simulink model "sgMdl_IO325_IO336_AnalogLoopback"  (R2024b)
settings: Solver=FixedStepAuto  StartTime=0.0  StopTime=inf  RelTol=1e-3
undefined symbols (not defined in the file): Pull, pull, up
libraries: speedgoatlib_fpga_analog_io x3, slrealtimeloglib x2, speedgoatlib_fpga x1
Description:
  | IO325 & IO336 - Analog Loopback
settings Model: ModifiedByFormat=Speedgoat  SimulationMode=external  ExtModeTrigDuration=100000  Creator=Speedgoat  LastModifiedBy=Speedgoat
settings SolverCC: ConcurrentTasks=on  PositivePriorityOrder=on
settings DataIOCC: SaveFormat=StructureWithTime
settings OptimizationCC: BlockReduction=off  OptimizeBlockIOStorage=off  BufferReuse=off  ReuseModelBlockBuffer=off
settings DebuggingCC: UnderspecifiedInitializationDetection=Classic  MergeDetectMultiDrivingBlocksExec=none  TasksWithSamePriorityMsg=none
settings HardwareCC: ProdBitPerLong=64  ProdLongLongMode=on  ProdHWDeviceType=Intel->x86-64 (Linux 64)
settings ModelReferenceCC: EnableRefExpFcnMdlSchedulingChecks=on  PropagateSignalLabelsOutOfModel=off
settings RTWCC: Description=Speedgoat Real-Time Target Machine  SystemTargetFile=speedgoat.tlc  TemplateMakefile=slrealtime_default_tmf  PostCodeGenCommand=sg.model.build.makeCfg(bdroot, buildInfo);  Toolchain=Simulink Real-Time Toolchain  BuildConfiguration=Faster Runs  TargetLang=C++  GPUComputeCapability=3.5
settings SimulinkRealTimeTargetCC: SubcomponentCodeInterfacePackaging=Reusable function  InstructionSetFMA=off  LogToMDFFile=off  SLRTFileLogMaxRuns=10
settings ConfigComp: CovBoundaryAbsTol=1.0e-5

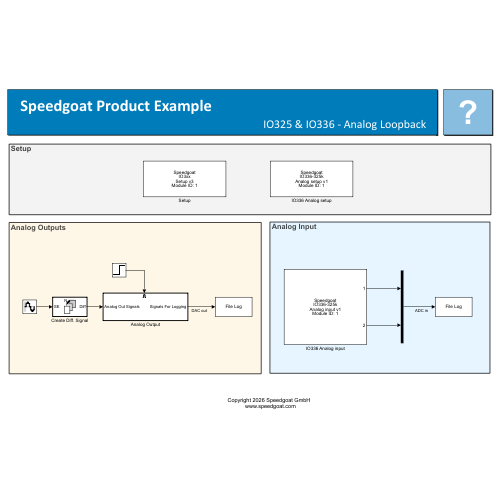
[thumbnail: Simulink's stored preview of the top-level diagram]
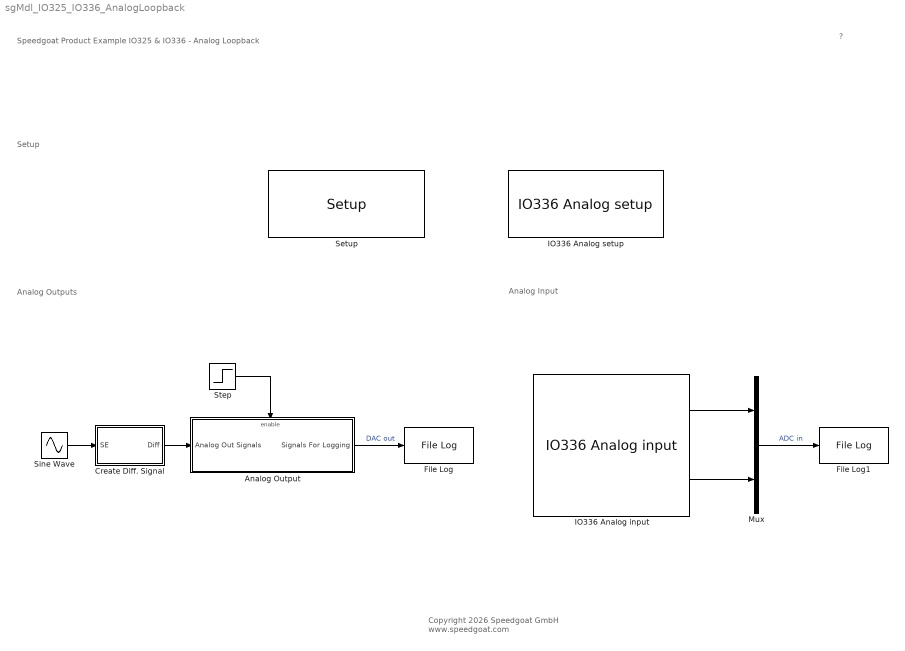
== system sgMdl_IO325_IO336_AnalogLoopback ==
  note: Analog Outputs
  note: Analog Input
  note: Setup
  note: Speedgoat Product Example
      | IO325 & IO336 - Analog Loopback
  note: ?
  note: Copyright 2026 Speedgoat GmbH
      |  www.speedgoat.com
  Analog Output : Subsystem
  Create Diff. Signal : Subsystem  TreatAsAtomicUnit=on
  File Log : slrealtimeloglib/File Log  decimation=1  inputProcessing=Elements as channels (sample based)
  File Log1 : slrealtimeloglib/File Log  decimation=1  inputProcessing=Elements as channels (sample based)
  IO336 Analog input : speedgoatlib_fpga_analog_io/IO336/IO336 Analog input  id=1  parSampleTime=1e-3  pciSlot=[-1,-1]  parAiChannels=[1 2]  parAiChannelsStreamed=[1 2]  parAiTriggerMode=[1 1]  parAiReadPrevValue=0  parAiEnableFrame=0  parAiVoltageRange=[0 3 3 3 3 3 3 3]  parAdcCoupling=[1 1 1 1]  parAdcContSampling=0  parAdcDmaEnable=0  parAdcActiveDmaDevices=[1 1 1 1]  parAiFrameSize=100
      settings: SourceProductName=Analog IO
  IO336 Analog setup : speedgoatlib_fpga_analog_io/IO336/IO336 Analog setup  id=1  parEnableCodeModule1=off  parEnableCodeModule2=off  parEnableCodeModule3=off  parEnableCodeModule4=off  parEnableCodeModule5=off  parEnableCodeModule6=off  parEnableCodeModule7=off  parEnableCodeModule8=off  parAdcEnableIndividualTrigger=off  parAdcTriggerMode1=Model Step  parAdcSampleRate1=0  parAdcDioTriggerChannel1=1  parAdcInternalTrigger1=<empty>  parAdcOversampling1=None  parAdcTriggerMode2=Model Step  parAdcSampleRate2=0  parAdcDioTriggerChannel2=1  parAdcInternalTrigger2=<empty>  parAdcOversampling2=None  parAdcReadPrevValueIndividualTrigger=off  parAdcEnableFrame=off  parAdcTriggerMode=Model Step  parAdcReadPrevValue=off  parAdcSampleRate=100e3  parAdcDioTriggerChannel=1  parAdcInternalTrigger=<empty>  parAdcOversampling=None  parAdcTriggerResolution=1e-08  parAdcSampleRateFrame=100e3  parAdcFrameSize=100  parAdcSampleTime=0.1  parDacTriggerMode=Model Step  parDacInternalTrigger=<empty>  parDacDioTriggerChannel=0  parDacEnableFrame=on  dacUsesTimer=on  parDacFifoThreshold=100  parDacTriggerResolution=1e-08  parDacSampleRate=1e6  parDacFrameSize=100  parDacSampleTime=0.1  parAdcChannel1=on  parAdcChannel2=on  parAdcChannel3=off  parAdcChannel4=off  parAdcChannel5=off  parAdcChannel6=off  parAdcChannel7=off  parAdcChannel8=off  parVoltageRangePerChannelEn1=off  parAdcRangeAll1=+/- 20V  parAdcRange1=+/- 20V  parAdcRange3=+/- 20V  parAdcRange2=+/- 20V  parAdcRange4=+/- 20V  parAdcChannel9=off  parAdcChannel10=off  parAdcChannel11=off  parAdcChannel12=off  parAdcChannel13=off  parAdcChannel14=off  parAdcChannel15=off  parAdcChannel16=off  parVoltageRangePerChannelEn2=off  parAdcRangeAll2=+/- 20V  parAdcRange5=+/- 20V  parAdcRange7=+/- 20V  parAdcRange6=+/- 20V  parAdcRange8=+/- 20V  parAdcAutoCorrection=on  parDacChannel1=on  parDacChannel2=on  parDacChannel3=on  parDacChannel4=on  parDacChannel5=off  parDacChannel6=off  parDacChannel7=off  parDacChannel8=off  parDacRange1=+-10 V  parDacInitValue1=0.5  parDacReset1=on  parDacRange2=+-10 V  parDacInitValue2=-0.5  parDacReset2=on  parDacRange3=+-10 V  parDacInitValue3=1  parDacReset3=on  parDacRange4=+-10 V  parDacInitValue4=-1  parDacReset4=on  parDacRange5=+-5 V  parDacInitValue5=0  parDacReset5=on  parDacRange6=+-5 V  parDacInitValue6=0  parDacReset6=on  parDacRange7=+-5 V  parDacInitValue7=0  parDacReset7=on  parDacRange8=+-5 V  parDacInitValue8=0  parDacReset8=on  parDacAutoCorrection=on
      settings: SourceProductName=Analog IO
  Mux : Mux  Inputs=2
  Setup : speedgoatlib_fpga/Setup/Setup  board=Please select...  id=1  pciSlot=-1  device_id=1  bitstreamFilePath=C:\SVN\speedgoatlib\releases\10.0.0\product_examples\IO325_IO336  bitstreamFile=Please select...  fpgaFreq=[100000000 100000000]  enableDma=on  rearEnb_1=off  rearIO_1=None  rearEnb_2=off  rearIO_2=None  ProgSpiFlash=off  ProgBPIFlash=off  useFpgaDmaController=off  dmaTrigDropdown=Model Step  dmaTrigSelect=0  dmaStopOnOverload=on  dmaModeSequential=on  dmaModeParallel=off  PullRPort15=pull-up 3.3V  PullRPort31=pull-up 3.3V  PullRPort47=pull-up 3.3V  PullRPort63=pull-up 3.3V  diffLineTermination_1=on  diffLineTermination_2=on  diffLineTermination_3=on  diffLineTermination_4=on  diffLineTermination_5=on  diffLineTermination_6=on  diffLineTermination_7=on  diffLineTermination_8=on  diffLineTermination_9=on  diffLineTermination_10=on  diffLineTermination_11=on  diffLineTermination_12=on  diffLineTermination_13=on  diffLineTermination_14=on  diffLineTermination_15=on  diffLineTermination_16=on  diffLineTermination_17=on  diffLineTermination_18=on  diffLineTermination_19=on  diffLineTermination_20=on  diffLineTermination_21=on  diffLineTermination_22=on  diffLineTermination_23=on  diffLineTermination_24=on  diffLineTermination_25=on  diffLineTermination_26=on  diffLineTermination_27=on  diffLineTermination_28=on  diffLineTermination_29=on  diffLineTermination_30=on  diffLineTermination_31=on  diffLineTermination_32=on  ioVoltageDropDown1=3.3V  pullResistorDropDown1_1=Pull-up  pullResistorDropDown1_2=Pull-up  pullResistorDropDown1_3=Pull-up  pullResistorDropDown1_4=Pull-up  pullResistorDropDown1_5=Pull-up  pullResistorDropDown1_6=Pull-up  pullResistorDropDown1_7=Pull-up  pullResistorDropDown1_8=Pull-up  ttlIsImplementedCheckBox1=off  pullResistorDropDown2=Pull-up  ioVoltageDropDown2=3.3V  ttlIsImplementedCheckBox2=off  pullResistorDropDown3=Pull-up  ioVoltageDropDown3=3.3V  ttlIsImplementedCheckBox3=off  pullResistorDropDown4=Pull-up  ioVoltageDropDown4=3.3V  ttlIsImplementedCheckBox4=off  pullResistorDropDown5=Pull-up  ioVoltageDropDown5=3.3V  ttlIsImplementedCheckBox5=off  pullResistorDropDown6=Pull-up  ioVoltageDropDown6=3.3V  ttlIsImplementedCheckBox6=off  pullResistorDropDown7=Pull-up  ioVoltageDropDown7=3.3V  ttlIsImplementedCheckBox7=off  pullResistorDropDown8=Pull-up  ioVoltageDropDown8=3.3V  ttlIsImplementedCheckBox8=off  terminationCheckBox1=off  terminationCheckBox2=off  terminationCheckBox3=off  terminationCheckBox4=off  diffIsImplementedCheckBox1=off  terminationCheckBox5=off  terminationCheckBox6=off  terminationCheckBox7=off  terminationCheckBox8=off  diffIsImplementedCheckBox2=off  terminationCheckBox9=off  terminationCheckBox10=off  terminationCheckBox11=off  terminationCheckBox12=off  diffIsImplementedCheckBox3=off  terminationCheckBox13=off  terminationCheckBox14=off  terminationCheckBox15=off  terminationCheckBox16=off  diffIsImplementedCheckBox4=off  terminationCheckBox17=off  terminationCheckBox18=off  terminationCheckBox19=off  terminationCheckBox20=off  diffIsImplementedCheckBox5=off  terminationCheckBox21=off  terminationCheckBox22=off  terminationCheckBox23=off  terminationCheckBox24=off  diffIsImplementedCheckBox6=off  terminationCheckBox25=off  terminationCheckBox26=off  terminationCheckBox27=off  terminationCheckBox28=off  diffIsImplementedCheckBox7=off  terminationCheckBox29=off  terminationCheckBox30=off  terminationCheckBox31=off  terminationCheckBox32=off  diffIsImplementedCheckBox8=off  PullRPort0_1=pull-up  VioPort0_1=3.3V  PullRPort1_1=pull-up  VioPort1_1=3.3V  PullRPort2_1=pull-up  VioPort2_1=3.3V  PullRPort3_1=pull-up  VioPort3_1=3.3V  PullRPort4_1=pull-up  VioPort4_1=3.3V  PullRPort5_1=pull-up  VioPort5_1=3.3V  PullRPort6_1=pull-up  VioPort6_1=3.3V  diffLineTermination_rear1_1=on  diffLineTermination_rear1_2=on  diffLineTermination_rear1_3=on  diffLineTermination_rear1_4=on  diffLineTermination_rear1_5=on  diffLineTermination_rear1_6=on  diffLineTermination_rear1_7=on  diffLineTermination_rear1_8=on  PullRPort0_2=pull-up  VioPort0_2=3.3V  PullRPort1_2=pull-up  VioPort1_2=3.3V  PullRPort2_2=pull-up  VioPort2_2=3.3V  PullRPort3_2=pull-up  VioPort3_2=3.3V  PullRPort4_2=pull-up  VioPort4_2=3.3V  PullRPort5_2=pull-up  VioPort5_2=3.3V  PullRPort6_2=pull-up  VioPort6_2=3.3V  diffLineTermination_rear2_1=on  diffLineTermination_rear2_2=on  diffLineTermination_rear2_3=on  diffLineTermination_rear2_4=on  diffLineTermination_rear2_5=on  diffLineTermination_rear2_6=on  diffLineTermination_rear2_7=on  diffLineTermination_rear2_8=on
      settings: SourceProductName=IO3xx
  Sine Wave : Sin  Amplitude=[1,2]  Frequency=10*2*pi  SampleTime=1e-3
  Step : Step  Time=0.5  SampleTime=1e-3
  wires:
  Mux/1 -> File Log1/1  "ADC in"
  IO336 Analog input/1 -> Mux/1
  IO336 Analog input/2 -> Mux/2
  Sine Wave/1 -> Create Diff. Signal/1(SE)
  Analog Output/1(Signals For Logging) -> File Log/1  "DAC out"
  Step/1 -> Analog Output/Enable
  Create Diff. Signal/1(Diff) -> Analog Output/1(Analog Out Signals)

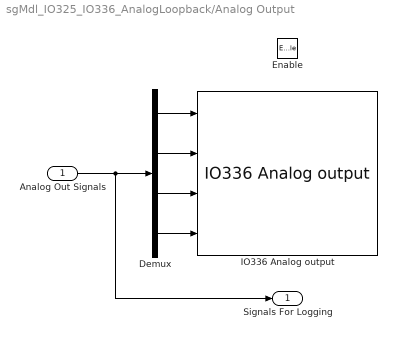
== system sgMdl_IO325_IO336_AnalogLoopback/Analog Output ==
  Analog Out Signals : Inport
  Enable : EnablePort
  Demux : Demux
  IO336 Analog output : speedgoatlib_fpga_analog_io/IO336/IO336 Analog output  id=1  parSampleTime=-1  pciSlot=[-1,-1]  board=Please select...  parAoChannels=[1 2 3 4]  parAoVoltageRange=[1 1 1 1]  parDacOverRange=[0 0 0 0 0 0 0 0]  parAoInitValues=[0.5 -0.5 1 -1]  parAoReset=[1 1 1 1]  parDacSyncOut=1  parAoEnableFrame=0  parDacActiveDmaDevices=[1 1 1 1]  parDacDmaLatency=2  parAoFrameSize=100
      settings: SourceProductName=Analog IO
  Signals For Logging : Outport
  wires:
  Demux/4 -> IO336 Analog output/4
  Analog Out Signals/1 -> Signals For Logging/1, Demux/1
  Demux/2 -> IO336 Analog output/2
  Demux/3 -> IO336 Analog output/3
  Demux/1 -> IO336 Analog output/1

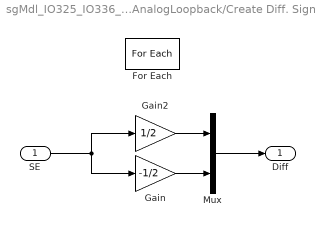
== system sgMdl_IO325_IO336_AnalogLoopback/Create Diff. Signal ==
  SE : Inport  Partition=on  PartitionDimension=1  PartitionWidth=1  PartitionOffset=0
  For Each : ForEach  DisableCoverage=on
  Gain : Gain  Gain=-1/2
  Gain2 : Gain  Gain=1/2
  Mux : Mux  Inputs=2
  Diff : Outport  ConcatenationDimension=1
  wires:
  Gain2/1 -> Mux/1
  Gain/1 -> Mux/2
  SE/1 -> Gain/1, Gain2/1
  Mux/1 -> Diff/1
